simulink model "PID_Controller"  (R2020b)
settings: Solver=VariableStepAuto  StartTime=0.0  StopTime=1  RelTol=1e-3
values from neighbouring files (symbols this model uses):
  Kd = 0.3    [motor_position_control_variable_data.sldd]
  Ki = 1500.0    [motor_position_control_variable_data.sldd]
  Kp = 100.0    [motor_position_control_variable_data.sldd]
  n = 1000000.0    [motor_position_control_variable_data.sldd]
settings Model: DataDictionary=motor_position_control_variable_data.sldd  Creator=dell  LastModifiedBy=dell
settings DataIOCC: SaveOutput=off  SaveTime=off

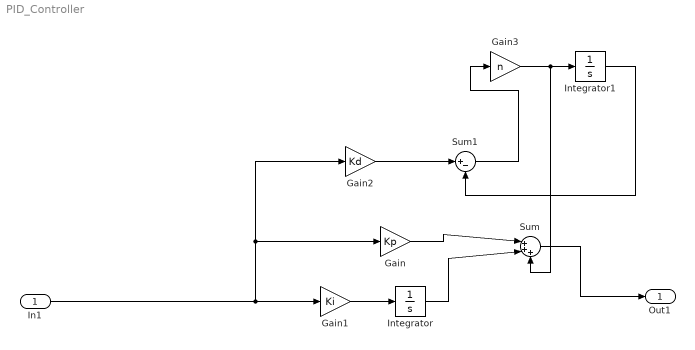
== system PID_Controller ==
  In1 : Inport  OutDataTypeStr=double  PortDimensions=1  SampleTime=0
  Gain : Gain  Gain=Kp
  Gain1 : Gain  Gain=Ki
  Gain2 : Gain  Gain=Kd
  Gain3 : Gain  Gain=n
  Integrator : Integrator
  Integrator1 : Integrator
  Sum : Sum  Inputs=|+++
  Sum1 : Sum  Inputs=|+-
  Out1 : Outport  OutDataTypeStr=double  PortDimensions=1  SampleTime=0
  wires:
  Sum/1 -> Out1/1
  In1/1 -> Gain/1, Gain2/1, Gain1/1
  Gain/1 -> Sum/1
  Gain1/1 -> Integrator/1
  Integrator/1 -> Sum/2
  Gain2/1 -> Sum1/1
  Integrator1/1 -> Sum1/2
  Gain3/1 -> Integrator1/1, Sum/3
  Sum1/1 -> Gain3/1
